simulink model "Q1"  (R2021a)
settings: Solver=FixedStepAuto  StartTime=0.0  StopTime=10  FixedStep=0.001  RelTol=1e-3
libraries: simulink x3
settings Model: Creator=M.M  LastModifiedBy=M.M

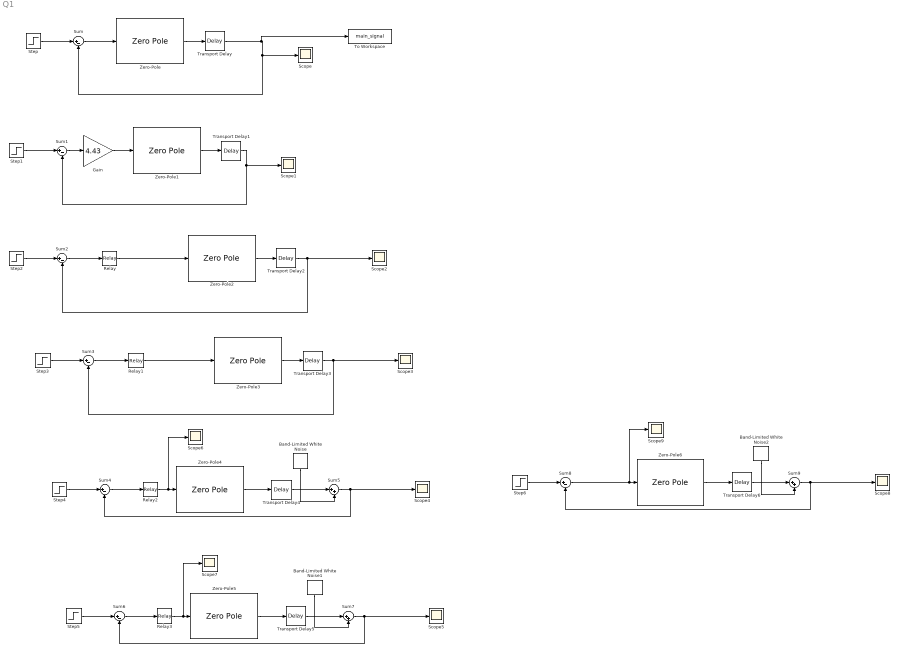
== system Q1 ==
  Band-Limited White Noise : simulink/Sources/Band-Limited White Noise  Cov=[0.01]  Ts=0.1  seed=[23341]
  Band-Limited White Noise1 : simulink/Sources/Band-Limited White Noise  Cov=[0.01]  Ts=0.1  seed=[23341]
  Band-Limited White Noise2 : simulink/Sources/Band-Limited White Noise  Cov=[0.01]  Ts=0.1  seed=[23341]
  Gain : Gain  Gain=4.43
  Relay : Relay  OffOutputValue=-1
  Relay1 : Relay  OffOutputValue=-1
  Relay2 : Relay  OffOutputValue=-1
  Relay3 : Relay  OnSwitchValue=0.05  OffSwitchValue=-0.05  OffOutputValue=-1
  Scope{,1..9} (10 alike) : Scope
  Step : Step  Time=0  SampleTime=0
  Step1 : Step  Time=0  SampleTime=0
  Step{2..6} (5 alike) : Step  Time=0  After=0  SampleTime=0
  Sum{,1..4,6,8} (7 alike) : Sum  Inputs=|+-
  Sum5 : Sum  Inputs=|++
  Sum7 : Sum  Inputs=|++
  Sum9 : Sum  Inputs=|++
  To Workspace : ToWorkspace  VariableName=main_signal  SaveFormat=Timeseries  SampleTime=-1
  Transport Delay{,1..6} (7 alike) : TransportDelay  DelayTime=0.1
  Zero-Pole{,1..6} (7 alike) : ZeroPole  Zeros=[-3]  Poles=[-2 -4]  Gain=[4]
  wires:
  Zero-Pole/1 -> Transport Delay/1
  Sum/1 -> Zero-Pole/1
  Step/1 -> Sum/1
  Transport Delay/1 -> To Workspace/1, Scope/1, Sum/2
  Zero-Pole1/1 -> Transport Delay1/1
  Transport Delay1/1 -> Scope1/1, Sum1/2
  Step1/1 -> Sum1/1
  Gain/1 -> Zero-Pole1/1
  Sum1/1 -> Gain/1
  Step2/1 -> Sum2/1
  Transport Delay2/1 -> Sum2/2, Scope2/1
  Relay/1 -> Zero-Pole2/1
  Zero-Pole2/1 -> Transport Delay2/1
  Sum2/1 -> Relay/1
  Relay1/1 -> Zero-Pole3/1
  Transport Delay3/1 -> Sum3/2, Scope3/1
  Step3/1 -> Sum3/1
  Sum3/1 -> Relay1/1
  Zero-Pole3/1 -> Transport Delay3/1
  Zero-Pole4/1 -> Transport Delay4/1
  Step4/1 -> Sum4/1
  Transport Delay4/1 -> Sum5/1
  Sum5/1 -> Scope4/1, Sum4/2
  Band-Limited White Noise/1 -> Sum5/2
  Relay2/1 -> Scope6/1, Zero-Pole4/1
  Sum4/1 -> Relay2/1
  Relay3/1 -> Scope7/1, Zero-Pole5/1
  Band-Limited White Noise1/1 -> Sum7/2
  Step5/1 -> Sum6/1
  Transport Delay5/1 -> Sum7/1
  Zero-Pole5/1 -> Transport Delay5/1
  Sum6/1 -> Relay3/1
  Sum7/1 -> Scope5/1, Sum6/2
  Sum8/1 -> Scope9/1, Zero-Pole6/1
  Band-Limited White Noise2/1 -> Sum9/2
  Step6/1 -> Sum8/1
  Transport Delay6/1 -> Sum9/1
  Zero-Pole6/1 -> Transport Delay6/1
  Sum9/1 -> Scope8/1, Sum8/2
